simulink model "ccmodel"  (R2023a)
settings: Solver=ode4  StartTime=0.0  StopTime=120  FixedStep=0.01  RelTol=1e-3
values from neighbouring files (symbols this model uses):
  b = cases(i,2)    [run_param.m]
  m = cases(i,1)    [run_param.m]
settings Model: Creator=sansh  LastModifiedBy=Fasih
settings SolverCC: AlgebraicLoopSolver=TrustRegion
settings DataIOCC: LoadExternalInput=on  ReturnWorkspaceOutputs=off
settings DebuggingCC: UnconnectedInputMsg=warning  UnconnectedOutputMsg=warning  UnconnectedLineMsg=warning  ArithmeticOperatorsInVariantConditions=warning
settings ModelReferenceCC: EnableRefExpFcnMdlSchedulingChecks=on
settings SFSimCC: SimUseLocalCustomCode=off  CustomCodeUndefinedFunction=UseInterfaceOnly
settings RTWCC: RTWUseLocalCustomCode=off
settings CodeAppCC: StateflowObjectComments=on

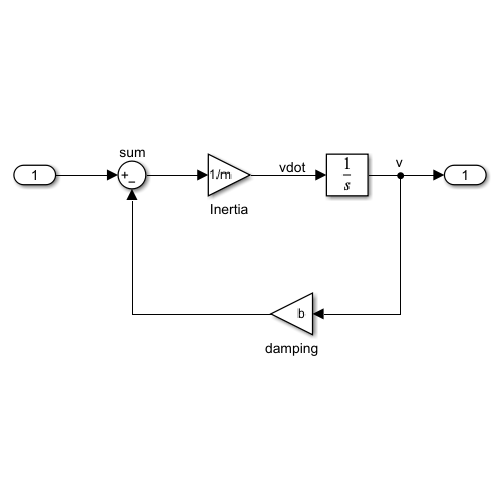
[thumbnail: Simulink's stored preview of the top-level diagram]
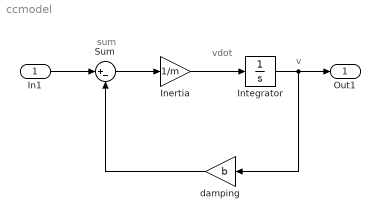
== system ccmodel ==
  note: v
  note: vdot
  note: sum
  In1 : Inport
  Inertia : Gain  Gain=1/m
  Integrator : Integrator
  Sum : Sum  Inputs=|+-
  damping : Gain  Gain=b
  Out1 : Outport
  wires:
  Integrator/1 -> Out1/1, damping/1
  Inertia/1 -> Integrator/1
  Sum/1 -> Inertia/1
  damping/1 -> Sum/2
  In1/1 -> Sum/1
